simulink model "test"  (R2017b)
settings: Solver=VariableStepAuto  StartTime=0.0  StopTime=2  MaxStep=1e-3  RelTol=1e-3
settings Model: Creator=lukasschwoerer  LastModifiedBy=lukasschwoerer

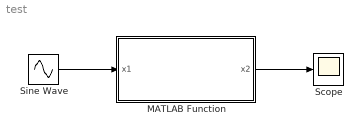
== system test ==
  MATLAB Function : MATLAB Function  TreatAsAtomicUnit=on
  Scope : Scope
  Sine Wave : Sin  Amplitude=2  Frequency=2*pi*1  SampleTime=0
  wires:
  Sine Wave/1 -> MATLAB Function/1(x1)
  MATLAB Function/1(x2) -> Scope/1

== matlab function test/MATLAB Function ==
  data: x1 input; x2 output
function x2 = kennlinie(x1)


%% Zone1 
if(x1<=0)
    x2 = 0;
else
    if(x1>=2)
        x2 = 3*x1 -6;
    else
        x2=2*sin(pi*x1);
    end
end
%% End
end
